simulink library "env_estimation_lib"  (R2016b)
settings: Solver=VariableStepAuto  StartTime=0.0  StopTime=10.0  RelTol=1e-3
libraries: ground_visualization x1, gs_prediction_lib x1, mag_vec_lib x1, sgp4_lib_fsw x1, sun_vector_lib x1, time_coord_rotation_lib x1
settings Model: Creator=taylorreynolds  LastModifiedBy=evich

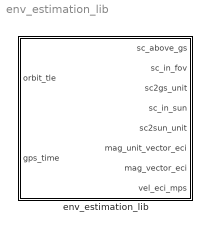
== system env_estimation_lib ==
  env_estimation_lib : Subsystem

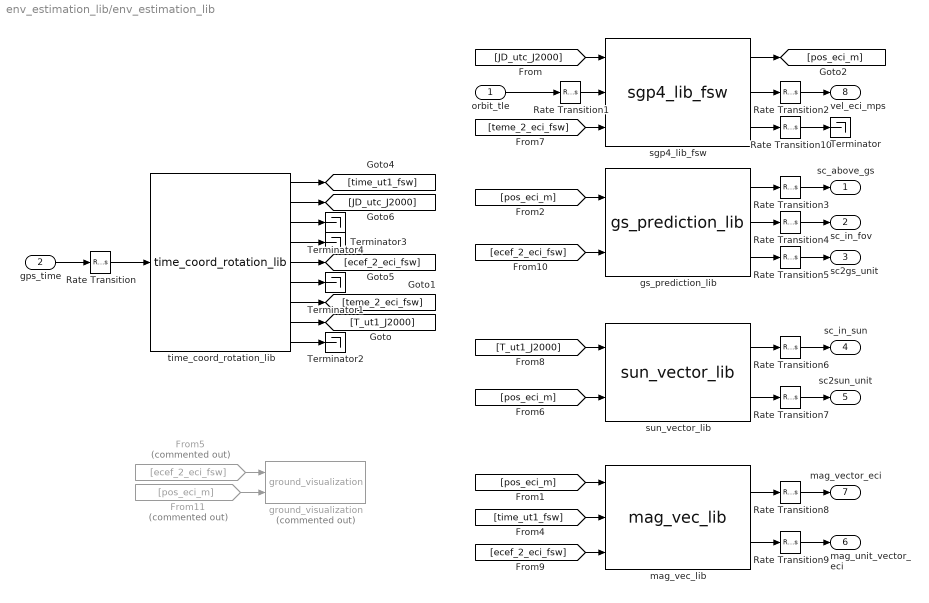
== system env_estimation_lib/env_estimation_lib ==
  orbit_tle : Inport
  gps_time : Inport  Port=2
  From11 : From  Commented=on  GotoTag=pos_eci_m
  From5 : From  Commented=on  GotoTag=ecef_2_eci_fsw
  Rate Transition : RateTransition  X0=fsw_params.env_estimation.ic.gps_time  OutPortSampleTime=fsw_params.env_estimation.sample_time_s
  Rate Transition1 : RateTransition  X0=fsw_params.env_estimation.ic.orbit_tle  OutPortSampleTime=fsw_params.env_estimation.sample_time_s
  Rate Transition{2..10} (9 alike) : RateTransition
  Terminator{,1..4} (5 alike) : Terminator
  ground_visualization : ground_visualization/ground_visualization  Commented=on
  gs_prediction_lib : gs_prediction_lib/gs_prediction_lib
  mag_vec_lib : mag_vec_lib/mag_vec_lib
  sgp4_lib_fsw : sgp4_lib_fsw/sgp4_lib_fsw
  sun_vector_lib : sun_vector_lib/sun_vector_lib
  time_coord_rotation_lib : time_coord_rotation_lib/time_coord_rotation_lib
  sc_above_gs : Outport
  sc_in_fov : Outport  Port=2
  sc2gs_unit : Outport  Port=3
  sc_in_sun : Outport  Port=4
  sc2sun_unit : Outport  Port=5
  mag_unit_vector_eci : Outport  Port=6
  mag_vector_eci : Outport  Port=7
  vel_eci_mps : Outport  Port=8
  wires:
  From11/1 -> ground_visualization/2
  From5/1 -> ground_visualization/1
  mag_vec_lib/2 -> Rate Transition9/1
  mag_vec_lib/1 -> Rate Transition8/1
  sun_vector_lib/2 -> Rate Transition7/1
  [T_ut1_J2000] -> sun_vector_lib/1
  [JD_utc_J2000] -> sgp4_lib_fsw/1
  [ecef_2_eci_fsw] -> mag_vec_lib/3
  [time_ut1_fsw] -> mag_vec_lib/2
  sun_vector_lib/1 -> Rate Transition6/1
  [pos_eci_m] -> sun_vector_lib/2
  [pos_eci_m] -> mag_vec_lib/1
  sgp4_lib_fsw/1 -> [pos_eci_m]
  orbit_tle/1 -> Rate Transition1/1
  gps_time/1 -> Rate Transition/1
  time_coord_rotation_lib/1 -> [time_ut1_fsw]
  gs_prediction_lib/1 -> Rate Transition3/1
  gs_prediction_lib/3 -> Rate Transition5/1
  gs_prediction_lib/2 -> Rate Transition4/1
  Rate Transition/1 -> time_coord_rotation_lib/1
  Rate Transition1/1 -> sgp4_lib_fsw/2
  Rate Transition2/1 -> vel_eci_mps/1
  Rate Transition3/1 -> sc_above_gs/1
  Rate Transition4/1 -> sc_in_fov/1
  Rate Transition5/1 -> sc2gs_unit/1
  Rate Transition6/1 -> sc_in_sun/1
  Rate Transition7/1 -> sc2sun_unit/1
  Rate Transition8/1 -> mag_vector_eci/1
  Rate Transition9/1 -> mag_unit_vector_eci/1
  [ecef_2_eci_fsw] -> gs_prediction_lib/2
  [pos_eci_m] -> gs_prediction_lib/1
  time_coord_rotation_lib/9 -> Terminator2/1
  time_coord_rotation_lib/8 -> [T_ut1_J2000]
  time_coord_rotation_lib/7 -> [teme_2_eci_fsw]
  time_coord_rotation_lib/6 -> Terminator1/1
  time_coord_rotation_lib/5 -> [ecef_2_eci_fsw]
  time_coord_rotation_lib/4 -> Terminator3/1
  time_coord_rotation_lib/3 -> Terminator4/1
  time_coord_rotation_lib/2 -> [JD_utc_J2000]
  [teme_2_eci_fsw] -> sgp4_lib_fsw/3
  sgp4_lib_fsw/2 -> Rate Transition2/1
  sgp4_lib_fsw/3 -> Rate Transition10/1
  Rate Transition10/1 -> Terminator/1
